simulink model "Proyecto_simulink"  (R2023a)
settings: Solver=VariableStepAuto  StartTime=0.0  StopTime=70.0  RelTol=1e-3
libraries: simulink x1
settings Model: Creator=pc  LastModifiedBy=pc

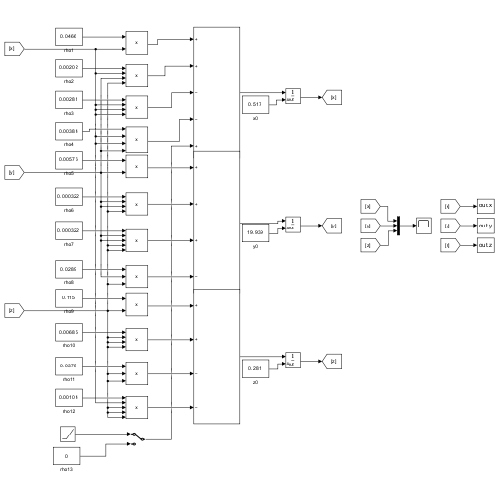
[thumbnail: Simulink's stored preview of the top-level diagram]
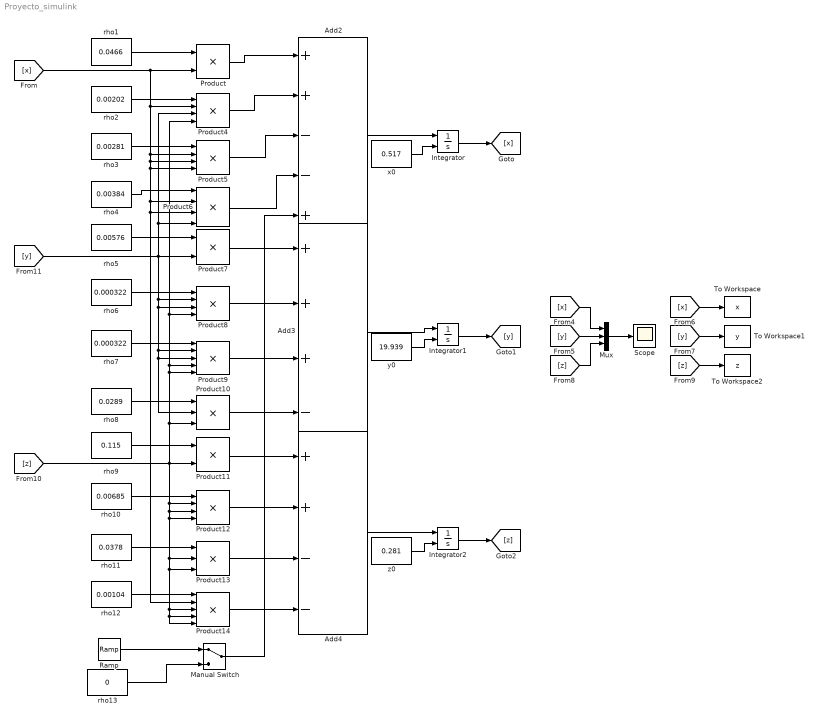
== system Proyecto_simulink ==
  Add2 : Sum  Inputs=++--+
  Add3 : Sum  Inputs=+++-
  Add4 : Sum  Inputs=++--
  Integrator : Integrator  InitialConditionSource=external
  Integrator1 : Integrator  InitialConditionSource=external
  Integrator2 : Integrator  InitialConditionSource=external
  Manual Switch : ManualSwitch
  Mux : Mux  Inputs=3
  Product : Product
  Product10 : Product  Inputs=3
  Product11 : Product
  Product{4..6,8,12} (5 alike) : Product  Inputs=4
  Product13 : Product  Inputs=3
  Product14 : Product  Inputs=5
  Product7 : Product
  Product9 : Product  Inputs=5
  Ramp : simulink/Sources/Ramp  slope=0.25  start=0  InitialOutput=0
  Scope : Scope
  To Workspace : ToWorkspace  VariableName=x  SampleTime=-1
  To Workspace1 : ToWorkspace  VariableName=y  SampleTime=-1
  To Workspace2 : ToWorkspace  VariableName=z  SampleTime=-1
  rho1 : Constant  Value=0.0466
  rho10 : Constant  Value=0.00685
  rho11 : Constant  Value=0.0378
  rho12 : Constant  Value=0.00104
  rho13 : Constant  Value=0
  rho2 : Constant  Value=0.00202
  rho3 : Constant  Value=0.00281
  rho4 : Constant  Value=0.00384
  rho5 : Constant  Value=0.00576
  rho6 : Constant  Value=0.000322
  rho7 : Constant  Value=0.000322
  rho8 : Constant  Value=0.0289
  rho9 : Constant  Value=0.115
  x0 : Constant  Value=0.517
  y0 : Constant  Value=19.939
  z0 : Constant  Value=0.281
  wires:
  [y] -> To Workspace1/1
  rho1/1 -> Product/1
  Integrator/1 -> [x]
  Mux/1 -> Scope/1
  Integrator1/1 -> [y]
  [y] -> Mux/2
  [x] -> To Workspace/1
  [x] -> Mux/1
  [z] -> Mux/3
  [z] -> To Workspace2/1
  [x] -> Product6/3, Product14/2, Product6/2, Product5/4, Product5/3, Product5/2, Product4/2, Product/2
  rho2/1 -> Product4/1
  rho3/1 -> Product5/1
  rho4/1 -> Product6/1
  rho5/1 -> Product7/1
  rho6/1 -> Product8/1
  rho7/1 -> Product9/1
  rho8/1 -> Product10/1
  rho9/1 -> Product11/1
  rho10/1 -> Product12/1
  rho11/1 -> Product13/1
  rho12/1 -> Product14/1
  [y] -> Product10/2, Product9/3, Product9/2, Product8/3, Product8/2, Product6/4, Product4/3, Product7/2
  [z] -> Product12/3, Product14/5, Product14/4, Product14/3, Product13/3, Product13/2, Product12/4, Product12/2, Product11/2, Product8/4, Product4/4, Product9/4, Product9/5, Product10/3
  Product/1 -> Add2/1
  Product4/1 -> Add2/2
  Product5/1 -> Add2/3
  Product6/1 -> Add2/4
  Product7/1 -> Add3/1
  Product8/1 -> Add3/2
  Product9/1 -> Add3/3
  Product10/1 -> Add3/4
  Product11/1 -> Add4/1
  Product13/1 -> Add4/3
  Product12/1 -> Add4/2
  Product14/1 -> Add4/4
  Integrator2/1 -> [z]
  Add4/1 -> Integrator2/1
  Add3/1 -> Integrator1/1
  Add2/1 -> Integrator/1
  x0/1 -> Integrator/2
  y0/1 -> Integrator1/2
  z0/1 -> Integrator2/2
  Manual Switch/1 -> Add2/5
  Ramp/1 -> Manual Switch/1
  rho13/1 -> Manual Switch/2
